simulink model "link3"  (R2016b)
settings: Solver=VariableStepAuto  StartTime=0.0  StopTime=10.0  RelTol=1e-3
settings Model: Creator=gz199  LastModifiedBy=gz199

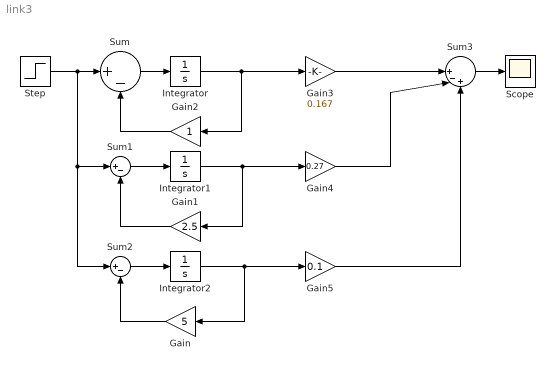
== system link3 ==
  Gain : Gain  Gain=5
  Gain1 : Gain  Gain=2.5
  Gain2 : Gain
  Gain3 : Gain  Gain=0.167
  Gain4 : Gain  Gain=0.27
  Gain5 : Gain  Gain=0.1
  Integrator : Integrator
  Integrator1 : Integrator
  Integrator2 : Integrator
  Scope : Scope
  Step : Step  Time=0  SampleTime=0
  Sum : Sum  Inputs=|+-
  Sum1 : Sum  Inputs=|+-
  Sum2 : Sum  Inputs=|+-
  Sum3 : Sum  Inputs=||+-+
  wires:
  Step/1 -> Sum2/1, Sum1/1, Sum/1
  Sum/1 -> Integrator/1
  Gain2/1 -> Sum/2
  Integrator2/1 -> Gain5/1, Gain/1
  Sum1/1 -> Integrator1/1
  Sum2/1 -> Integrator2/1
  Gain/1 -> Sum2/2
  Gain1/1 -> Sum1/2
  Sum3/1 -> Scope/1
  Integrator1/1 -> Gain1/1, Gain4/1
  Integrator/1 -> Gain2/1, Gain3/1
  Gain3/1 -> Sum3/1
  Gain4/1 -> Sum3/2
  Gain5/1 -> Sum3/3
